simulink model "ConvertisseurSigmaDelta"  (R2023a)
settings: Solver=VariableStepAuto  StartTime=0.0  StopTime=Tsim  FixedStep=TsR  RelTol=1e-3  EnableMultiTasking=on
values from neighbouring files (symbols this model uses):
  Ts = 1/nus    [CANSurechantillonnage.m]    (also in mConvertisseurSigmaDelta.m; mModulateurSigmaDelta.m)
  TsR = 1/nusR    [CANSurechantillonnage.m]    (also in mConvertisseurSigmaDelta.m = Ts/R; mModulateurSigmaDelta.m = Ts/R)
undefined symbols (not defined in the file or in its folder): A, B, gk, nu0
settings Model: ExtModeTrigMode=oneshot  Creator=gscorlet  LastModifiedBy=arthur.perodou
settings SolverCC: AlgebraicLoopSolver=TrustRegion
settings DataIOCC: SaveFormat=Array  SignalLoggingSaveFormat=ModelDataLogs  ReturnWorkspaceOutputs=off
settings OptimizationCC: BlockReduction=off  BooleanDataType=off  ReuseModelBlockBuffer=off  ExpressionDepthLimit=2147483647  LifeSpan=inf
settings DebuggingCC: SaveWithParameterizedLinksMsg=none  UnderspecifiedInitializationDetection=Classic  MergeDetectMultiDrivingBlocksExec=none  SignalResolutionControl=TryResolveAllWithWarning  MultiTaskDSMMsg=warning  MultiTaskCondExecSysMsg=none  FcnCallInpInsideContextMsg=warning  UnconnectedInputMsg=warning  UnconnectedOutputMsg=warning  UnconnectedLineMsg=warning  StateNameClashWarn=warning  SFUnexpectedBacktrackingDiag=warning  SFNoUnconditionalDefaultTransitionDiag=warning  SFExecutionAtInitializationDiag=none  ArithmeticOperatorsInVariantConditions=warning
settings HardwareCC: ProdBitPerPointer=32  ProdBitPerSizeT=32  ProdBitPerPtrDiffT=32  ProdLargestAtomicFloat=None  ProdIntDivRoundTo=Undefined  ProdEndianess=Unspecified  ProdWordSize=32  ProdHWDeviceType=32-bit Generic  TargetUnknown=on
settings ModelReferenceCC: PropagateSignalLabelsOutOfModel=off
settings SFSimCC: SimUseLocalCustomCode=off  CustomCodeUndefinedFunction=UseInterfaceOnly
settings RTWCC: RTWUseLocalCustomCode=off
settings CodeAppCC: StateflowObjectComments=on
settings GRTTargetCC: TargetLangStandard=C89/C90 (ANSI)  CombineOutputUpdateFcns=off  GRTInterface=on
settings ConfigComp: CovMetricSettings=dw  CovSaveCumulativeToWorkspaceVar=on  CovSaveSingleToWorkspaceVar=on  CovExternalEMLEnable=off  CovBoundaryAbsTol=1.0e-5

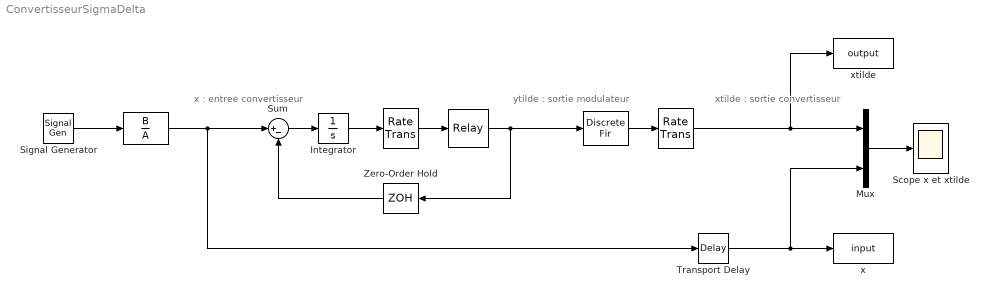
== system ConvertisseurSigmaDelta ==
  note: x : entree
      | convertisseur
  note: ytilde : sortie
      | modulateur
  note: xtilde : sortie
      | convertisseur
  " " : TransferFcn  Numerator=B  Denominator=A
  "  " : RateTransition  OutPortSampleTime=TsR
  "   " : Relay  OffSwitchValue=-eps  OffOutputValue=-1
  "    " : DiscreteFir  Coefficients=gk
  "      " : RateTransition  OutPortSampleTime=Ts
  Integrator : Integrator
  Mux : Mux  Inputs=2
  Scope x et xtilde : Scope
  Signal Generator : SignalGenerator  Frequency=nu0
  Sum : Sum  Inputs=|+-  InputSameDT=on  SaturateOnIntegerOverflow=on  OutDataTypeStr=Inherit: Same as first input
  Transport Delay : TransportDelay  DelayTime=1*Ts
  Zero-Order Hold : ZeroOrderHold  SampleTime=-1
  x : ToWorkspace  VariableName=input  SaveFormat=Timeseries  SampleTime=TsR
  xtilde : ToWorkspace  VariableName=output  SaveFormat=Timeseries  SampleTime=-1
  wires:
  Integrator/1 -> "  "/1
  Sum/1 -> Integrator/1
  Signal Generator/1 -> " "/1
  Mux/1 -> Scope x et xtilde/1
  "  "/1 -> "   "/1
  "   "/1 -> Zero-Order Hold/1, "    "/1
  "    "/1 -> "      "/1
  Transport Delay/1 -> x/1, Mux/2
  "      "/1 -> Mux/1, xtilde/1
  Zero-Order Hold/1 -> Sum/2
  " "/1 -> Transport Delay/1, Sum/1
